simulink model "demo_model"  (R2022b)
settings: Solver=VariableStepAuto  StartTime=0.0  StopTime=10.0  RelTol=1e-3
values from neighbouring files (symbols this model uses):
  K_lqr = [-0.244152194552 1.77852805994 -0.0833080959801 0.160626353487]    [model_greyest.mat]
  k_r_lqr = 1/k_dc_lqr    [demo_greyest.m]
  sys_qube_upright = ss(A_upright_d,B_upright_d,sys.C,sys.D,Ts)    [demo_greyest.m]
libraries: mpclib x1
settings Model: Creator=tonytang  LastModifiedBy=tonytang
settings DebuggingCC: UnconnectedInputMsg=warning  UnconnectedOutputMsg=warning  UnconnectedLineMsg=warning
settings ModelReferenceCC: EnableRefExpFcnMdlSchedulingChecks=on
settings RTWCC: DLArmComputeVersion=19.05

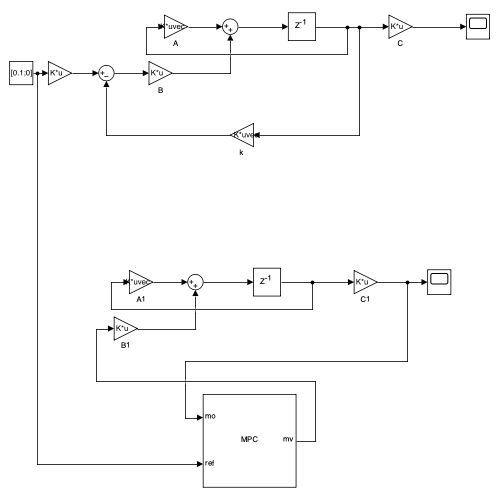
[thumbnail: Simulink's stored preview of the top-level diagram]
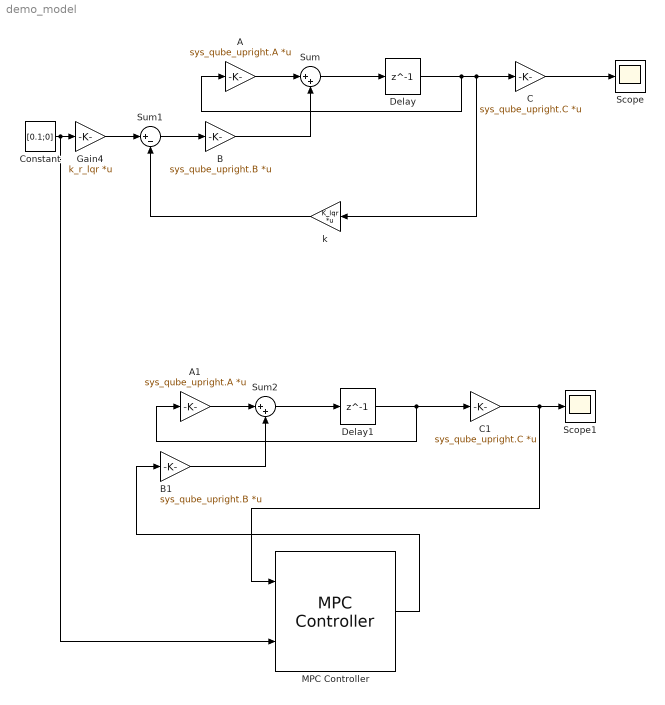
== system demo_model ==
  A : Gain  Gain=sys_qube_upright.A  Multiplication=Matrix(K*u) (u vector)
  A1 : Gain  Gain=sys_qube_upright.A  Multiplication=Matrix(K*u) (u vector)
  B : Gain  Gain=sys_qube_upright.B  Multiplication=Matrix(K*u)
  B1 : Gain  Gain=sys_qube_upright.B  Multiplication=Matrix(K*u)
  C : Gain  Gain=sys_qube_upright.C  Multiplication=Matrix(K*u)
  C1 : Gain  Gain=sys_qube_upright.C  Multiplication=Matrix(K*u)
  Constant : Constant  Value=[0.1;0]
  Delay : Delay  DelayLength=1  InitialCondition=[0;0;0;0]  SampleTime=0.01
  Delay1 : Delay  DelayLength=1  InitialCondition=[0;0;0;0]  SampleTime=0.01
  Gain4 : Gain  Gain=k_r_lqr  Multiplication=Matrix(K*u)
  MPC Controller : mpclib/MPC Controller  SCDEnableBlockLinearizationSpecification=on  mpcobj=mpcobj  x0=[]  is_multiple=0  enable_value=0  return_u0=off  updateMPCinCallerWorkspace=on  md_inport=off  mv_inport=off  uref_inport=off  return_cost=off  return_mvseq=off  return_qpstatus=off  return_xseq=off  return_state=off  return_ovseq=off  state_inport=off  umin_inport=off  umax_inport=off  ymin_inport=off  ymax_inport=off  cc_inport=off  ywt_inport=off  uwt_inport=off  duwt_inport=off  rhoeps_inport=off  pm_inport=off  MaximumP=10  HorizonChoice=FixedHorizon  n_ts=0.01  n_p=10  n_mv=1  n_md=1  n_ud=0  n_mo=2  n_uo=0  BlockDataType=double  SampleTimeInherited=off  switch_inport=off
  Scope : Scope
  Scope1 : Scope
  Sum : Sum  Inputs=|++
  Sum1 : Sum  Inputs=|+-
  Sum2 : Sum  Inputs=|++
  k : Gain  Gain=K_lqr  Multiplication=Matrix(K*u) (u vector)
  wires:
  Delay/1 -> A/1, k/1, C/1
  C/1 -> Scope/1
  Sum/1 -> Delay/1
  A/1 -> Sum/1
  B/1 -> Sum/2
  k/1 -> Sum1/2
  Constant/1 -> MPC Controller/2, Gain4/1
  Gain4/1 -> Sum1/1
  Sum1/1 -> B/1
  Sum2/1 -> Delay1/1
  Delay1/1 -> A1/1, C1/1
  C1/1 -> Scope1/1, MPC Controller/1
  MPC Controller/1 -> B1/1
  A1/1 -> Sum2/1
  B1/1 -> Sum2/2
